simulink subsystem "full_controller_frictionComp"  (R2022a)
settings: Solver=VariableStepAuto  StartTime=0.0  StopTime=10.0  RelTol=1e-3
settings Model: Creator=Philipp  LastModifiedBy=Philipp

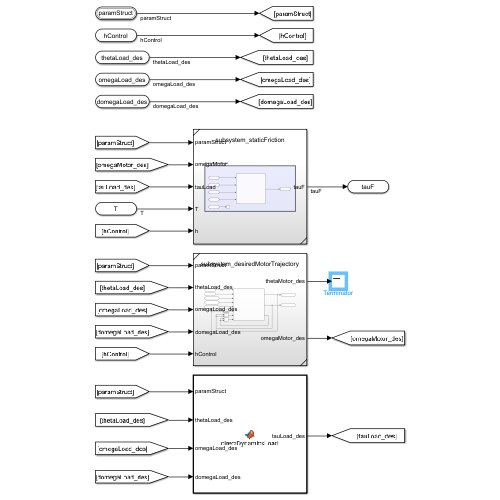
[thumbnail: Simulink's stored preview of the top-level diagram]
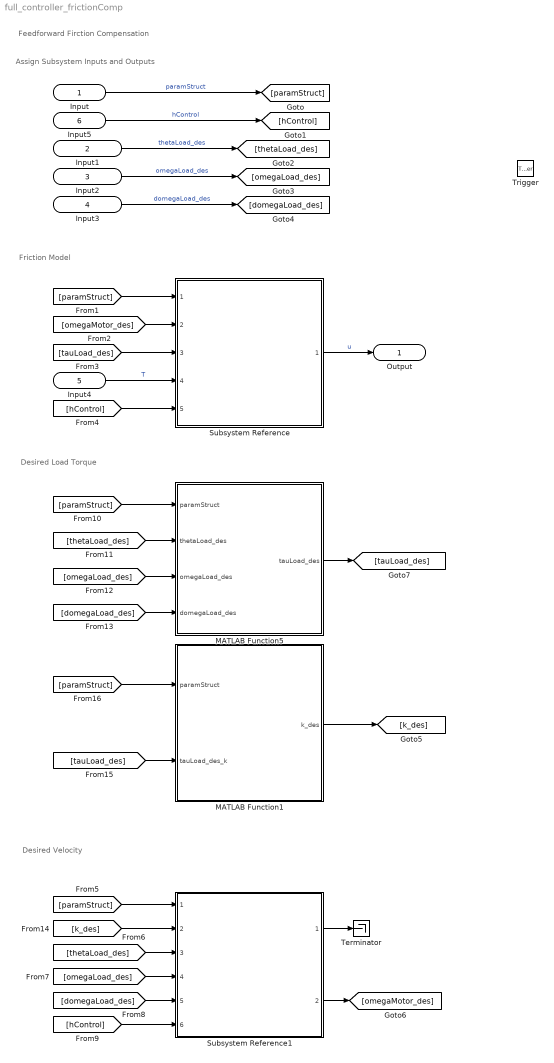
== system full_controller_frictionComp ==
  note: Desired Velocity
  note: Desired Load Torque
  note: Friction Model
  note: Assign Subsystem Inputs and Outputs
  note: Feedforward Firction Compensation
  Input : Inport  OutDataTypeStr=Bus: main_bus
  Input1 : Inport  Port=2
  Input2 : Inport  Port=3
  Input3 : Inport  Port=4
  Input4 : Inport  Port=5
  Input5 : Inport  Port=6
  Trigger : TriggerPort  VariantControl=(inherit)
  MATLAB Function1 : MATLAB Function  TreatAsAtomicUnit=on
  MATLAB Function5 : MATLAB Function  TreatAsAtomicUnit=on
  Subsystem Reference : Subsystem  ReferencedSubsystem=subsystem_lugreFriction
  Subsystem Reference1 : Subsystem  ReferencedSubsystem=subsystem_desiredMotorTrajectory
  Terminator : Terminator
  Output : Outport
  wires:
  Subsystem Reference/1 -> Output/1  "u"
  [domegaLoad_des] -> Subsystem Reference1/5
  [hControl] -> Subsystem Reference1/6
  [paramStruct] -> Subsystem Reference1/1
  [omegaLoad_des] -> Subsystem Reference1/4
  [thetaLoad_des] -> Subsystem Reference1/3
  Subsystem Reference1/1 -> Terminator/1
  Subsystem Reference1/2 -> [omegaMotor_des]
  Input/1 -> [paramStruct]  "paramStruct"
  Input5/1 -> [hControl]  "hControl"
  [paramStruct] -> Subsystem Reference/1
  [omegaMotor_des] -> Subsystem Reference/2
  [tauLoad_des] -> Subsystem Reference/3
  Input4/1 -> Subsystem Reference/4  "T"
  [hControl] -> Subsystem Reference/5
  Input3/1 -> [domegaLoad_des]  "domegaLoad_des"
  Input2/1 -> [omegaLoad_des]  "omegaLoad_des"
  Input1/1 -> [thetaLoad_des]  "thetaLoad_des"
  [paramStruct] -> MATLAB Function5/1(paramStruct)
  [thetaLoad_des] -> MATLAB Function5/2(thetaLoad_des)
  [omegaLoad_des] -> MATLAB Function5/3(omegaLoad_des)
  [domegaLoad_des] -> MATLAB Function5/4(domegaLoad_des)
  MATLAB Function5/1(tauLoad_des) -> [tauLoad_des]
  [k_des] -> Subsystem Reference1/2
  [tauLoad_des] -> MATLAB Function1/2(tauLoad_des_k)
  [paramStruct] -> MATLAB Function1/1(paramStruct)
  MATLAB Function1/1(k_des) -> [k_des]

== matlab function full_controller_frictionComp/MATLAB Function1 ==
  data: k_des output; paramStruct input; tauLoad_des_k input
function k_des  = stiffness_des(paramStruct, tauLoad_des_k)

c_k = paramStruct.robot.c_k;

% Calculate desired stiffness
kDeg_des = stiffnessTauE(c_k, tauLoad_des_k);

% Convert to rad
k_des = kDeg_des .* (180/pi);

== matlab function full_controller_frictionComp/MATLAB Function5 ==
  data: paramStruct input; thetaLoad_des input; tauLoad_des output; omegaLoad_des input; domegaLoad_des input
function tauLoad_des = directDynamicsLoad(paramStruct, thetaLoad_des, omegaLoad_des, domegaLoad_des)

g = paramStruct.robot.g;
r_P1P2 = paramStruct.robot.r_P1P2;
r_P2P3 = paramStruct.robot.r_P2P3;
r_P3P4 = paramStruct.robot.r_P3P4;
baseParam = paramStruct.robot.baseParam;

tauLoad_des = ...
    inverseDynamics_rigid_fun(g, r_P1P2, r_P2P3, r_P3P4, baseParam, thetaLoad_des, omegaLoad_des, domegaLoad_des, zeros(3,1));
